simulink model "ESP_Model"  (R2021a)
settings: Solver=VariableStepAuto  StartTime=0.0  StopTime=30.0  MaxStep=1e-3  RelTol=1e-3
values from neighbouring files (symbols this model uses):
  C1 = [0 1]    [Main.m]
  C2 = C1    [Main.m]
  deltaFront = 0*[1 1 0 0]/180*pi    [Main.m]
  H = [ones(1,4) ... (first row only)    [Main.m]
  lambda0s = fsolve(f,0)    [Main.m]
  pinv_de_tau = pinv(de_tau)    [Main.m]
  v0 = 130/3.6    (= 36.1111111111)    [Main.m]
undefined symbols (not defined in the file or in its folder): Kr, u_tilde, xr_dot
settings Model: Creator=patta  LastModifiedBy=atavo
settings SolverCC: AlgebraicLoopSolver=TrustRegion
settings DataIOCC: ReturnWorkspaceOutputs=off
settings DebuggingCC: SFMachineParentedDataDiag=warning  ArithmeticOperatorsInVariantConditions=warning
settings SFSimCC: CustomCodeUndefinedFunction=UseInterfaceOnly

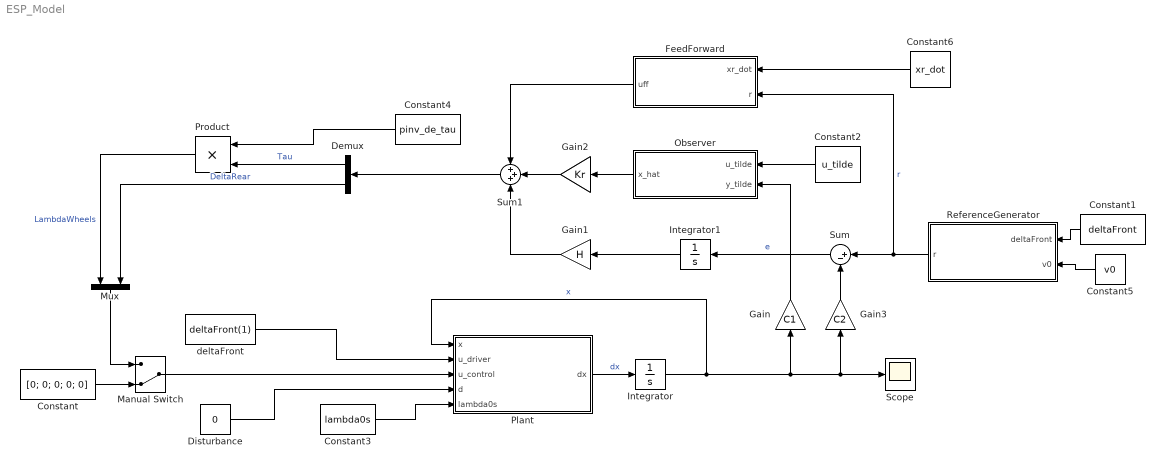
== system ESP_Model ==
  Constant : Constant  Value=[0; 0; 0; 0; 0]
  Constant1 : Constant  Value=deltaFront
  Constant2 : Constant  Value=u_tilde
  Constant3 : Constant  Value=lambda0s
  Constant4 : Constant  Value=pinv_de_tau
  Constant5 : Constant  Value=v0
  Constant6 : Constant  Value=xr_dot
  Demux : Demux  Outputs=2
  Disturbance : Constant  Value=0
  FeedForward : MATLAB Function  TreatAsAtomicUnit=on
  Gain : Gain  Gain=C1
  Gain1 : Gain  Gain=H
  Gain2 : Gain  Gain=Kr
  Gain3 : Gain  Gain=C2
  Integrator : Integrator  InitialCondition=[5; 0]
  Integrator1 : Integrator
  Manual Switch : ManualSwitch  CurrentSetting=0
  Mux : Mux  Inputs=2
  Observer : MATLAB Function  TreatAsAtomicUnit=on
  Plant : MATLAB Function  TreatAsAtomicUnit=on
  Product : Product
  ReferenceGenerator : MATLAB Function  TreatAsAtomicUnit=on
  Scope : Scope
  Sum : Sum  Inputs=|+-
  Sum1 : Sum  Inputs=+++
  deltaFront : Constant  Value=deltaFront(1)
  wires:
  Plant/1(dx) -> Integrator/1  "dx"
  Integrator/1 -> Plant/1(x), Gain/1, Gain3/1, Scope/1  "x"
  deltaFront/1 -> Plant/2(u_driver)
  Disturbance/1 -> Plant/4(d)
  Constant3/1 -> Plant/5(lambda0s)
  Constant4/1 -> Product/1
  Demux/1 -> Product/2  "Tau"
  Product/1 -> Mux/1  "LambdaWheels"
  Demux/2 -> Mux/2  "DeltaRear"
  Mux/1 -> Manual Switch/1
  Constant/1 -> Manual Switch/2
  Manual Switch/1 -> Plant/3(u_control)
  Observer/1(x_hat) -> Gain2/1
  Gain2/1 -> Sum1/2
  Sum/1 -> Integrator1/1  "e"
  Integrator1/1 -> Gain1/1
  Constant1/1 -> ReferenceGenerator/1(deltaFront)
  Constant2/1 -> Observer/1(u_tilde)
  Gain1/1 -> Sum1/3
  FeedForward/1(uff) -> Sum1/1
  Sum1/1 -> Demux/1
  Gain/1 -> Observer/2(y_tilde)
  Gain3/1 -> Sum/2
  ReferenceGenerator/1(r) -> FeedForward/2(r), Sum/1  "r"
  Constant5/1 -> ReferenceGenerator/2(v0)
  Constant6/1 -> FeedForward/1(xr_dot)

== matlab function ESP_Model/ReferenceGenerator ==
  data: r output; deltaFront input; v0 input
function r = ReferenceGenerator(deltaFront,v0)

delta_f = (deltaFront(1)+deltaFront(2))/2;

g = 9.81; % [m/s^2] gravity acceleration
rho = 1.225; % [kg/m^3] air density
S = 2.4; % [m^2] cross surface
Cx0 = -0.3; % [-] drag coefficient
Cyb = -0.3; % [-] drag coefficient

m = 1200; % [kg] vehicle mass
rxf = 1.4;
rxr = -1.6;
ryf = 0.90;
Iz = 1200*(rxr^2+ryf^2)^2;
rx = [rxf rxf rxr rxr];
ry = [ryf -ryf -ryf ryf];
rz =  0.70;

H = [ones(1,4);
    ry;
    -rx];


beta0 = 0;
w0 = 0;
theta = 0/180*pi;

pinvH = pinv(H);
FzW = pinvH*(rz/2*rho*S*v0^2*[0; Cyb*sin(beta0); -Cx0*cos(beta0)]+[m*g*cos(theta); -rz*m*v0*w0*cos(beta0); -rz*m*g*sin(theta)-rz*m*v0*w0*sin(beta0)]);
Cf = (FzW(1)+FzW(2))*Partial_mu_long(1,0);
Cr = (FzW(3)+FzW(4))*Partial_mu_long(1,0);

A11 = -(Cf+Cr)/(m*v0);
A12 = -v0-(Cf*rxf+Cr*rxr)/(m*v0);
A21 = -(Cf*rxf+Cr*rxr)/(Iz*v0);
A22 = -(Cf*rxf^2+Cr*rxr^2)/(Iz*v0);
A = [A11 A12
     A21 A22];
B1 = Cf*[1/m;
      rxf/Iz];

function mu = Partial_mu_long(i,lambda)

% 1) Dry asphalt
% 2) wet asphalt
% 3) Snow
% 4) Ice
% 5) Dry Cobblestone
% 6) wet cobblestone
theta1 = [1.28 0.86 0.19 0.05 1.37 0.4];
theta2 = [23.99 33.82 94.13 306.39 6.46 33.71];
theta3 = [0.52 0.35 0.05 0 0.67 0.12];

mu = theta1(i).*theta2(i).*exp(-abs(lambda).*theta2(i))-theta3(i);

end


r = -inv(A)*B1*delta_f;

== matlab function ESP_Model/Plant ==
  data: x input; dx output; u_driver input; u_control input; d input; lambda0s input
function dx = Plant(x,u_driver,u_control,d, lambda0s)

g = 9.81; % [m/s^2] gravity acceleration
rho = 1.225; % [kg/m^3] air density
S = 2.4; % [m^2] cross surface
Cx0 = -0.3; % [-] drag coefficient
Cyb = -0.3; % [-] drag coefficient
rk = 1; % dry asphalt
m = 1200; % [kg] vehicle mass
rxf = 1.4;
rxr = -0.5;
ryf = 0.90;
rz =  0.70;
CR = -0.05;
Iz = 1200*(rxr^2 + ryf^2)^2;

delta = 0*[1 1 0 0]/180*pi; % 3.5 // 10

rx = [rxf rxf rxr rxr];
ry = [ryf -ryf -ryf ryf];
H = [ones(1,4);
    ry;
    -rx];

%% EQUILIBRIUM POINT

%  global v0 FzW

x0 = 0;
y0 = 0;
v0 = 270/3.6; % [m/s] vehicle speed
beta0 = 0;
w0 = 0;
psi0 = 0/180*pi;
theta = 15/180*pi;

pinvH = pinv(H);
FzW = pinvH*(rz/2*rho*S*v0^2*[0; Cyb*sin(beta0); -Cx0*cos(beta0)]+[m*g*cos(theta); -rz*m*v0*w0*cos(beta0); -rz*m*g*sin(theta)-rz*m*v0*w0*sin(beta0)]);

lambda0s = 0.0061;  %found in main
lambda0 = [lambda0s; lambda0s; 0; 0];

Cf = (FzW(1)+FzW(2))*Partial_mu_long(1,0);
Cr = (FzW(3)+FzW(4))*Partial_mu_long(1,0);
A11 = -(Cf+Cr)/(m*v0);
A12 = -v0-(Cf*rxf+Cr*rxr)/(m*v0);
A21 = -(Cf*rxf+Cr*rxr)/(Iz*v0);
A22 = -(Cf*rxf^2+Cr*rxr^2)/(Iz*v0);
A = [A11 A12
    A21 A22];
B1 = Cf*[1/m;
      rxf/Iz];
B1_Ctrl = [zeros(1,4) Cr*(1/m);
             (FzW.').*[(ryf/Iz)*(-Partial_mu_long(1,lambda0s)) (ryf/Iz)*(Partial_mu_long(1,lambda0s)) (ryf/Iz)*(Partial_mu_long(1,0)) (ryf/Iz)*(-Partial_mu_long(1,0))] Cr*(rxr/Iz)];
B2eq = [0; 1/Iz];

dx = A*x+B1*u_driver+B1_Ctrl*u_control;

end

%% Mu

function mu = mu_long(i,lambda)

% 1) Dry asphalt
% 2) wet asphalt
% 3) Snow
% 4) Ice
% 5) Dry Cobblestone
% 6) wet cobblestone
theta1 = [1.28 0.86 0.19 0.05 1.37 0.4];
theta2 = [23.99 33.82 94.13 306.39 6.46 33.71];
theta3 = [0.52 0.35 0.05 0 0.67 0.12];

mu = sign(lambda).*theta1(i).*(1-exp(-abs(lambda)*theta2(i)))-theta3(i)*lambda;

end

%%Partial derivative of mu

function mu = Partial_mu_long(i,lambda)

% 1) Dry asphalt
% 2) wet asphalt
% 3) Snow
% 4) Ice
% 5) Dry Cobblestone
% 6) wet cobblestone
theta1 = [1.28 0.86 0.19 0.05 1.37 0.4];
theta2 = [23.99 33.82 94.13 306.39 6.46 33.71];
theta3 = [0.52 0.35 0.05 0 0.67 0.12];

mu = theta1(i).*theta2(i).*exp(-abs(lambda).*theta2(i))-theta3(i);

end

== matlab function ESP_Model/Observer ==
  data: u_tilde input; y_tilde input; x_hat output
function x_hat = Observer(u_tilde, y_tilde)

x_hat = u;

== matlab function ESP_Model/FeedForward ==
  data: xr_dot input; r input; uff output
function uff = FeedForward(xr_dot, r)






uff = inv((C2*inv(A + B1_Ctrl*Kr))*B1_Ctrl)*(r + C2*inv(A + B1_Ctrl*Kr)*xr_dot;
